simulink model "sampleModel1976_1_sub_sub"  (R2023a)
settings: Solver=VariableStepAuto  StartTime=0.0  StopTime=10.0  RelTol=1e-3
libraries: hdlsllib x5, simulink x1
settings Model: Creator=user1  LastModifiedBy=user1
settings OptimizationCC: BlockReduction=off  ConditionallyExecuteInputs=off

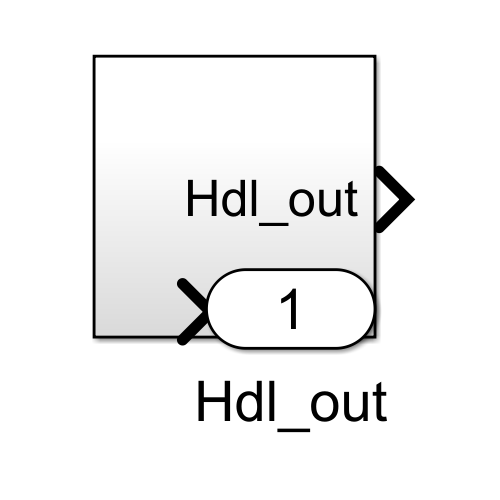
[thumbnail: Simulink's stored preview of the top-level diagram]
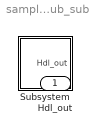
== system sampleModel1976_1_sub_sub ==
  Subsystem : Subsystem
  Hdl_out : Outport  OutDataTypeStr=uint8

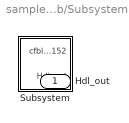
== system sampleModel1976_1_sub_sub/Subsystem ==
  Subsystem : Subsystem
  Hdl_out : Outport  OutDataTypeStr=uint8

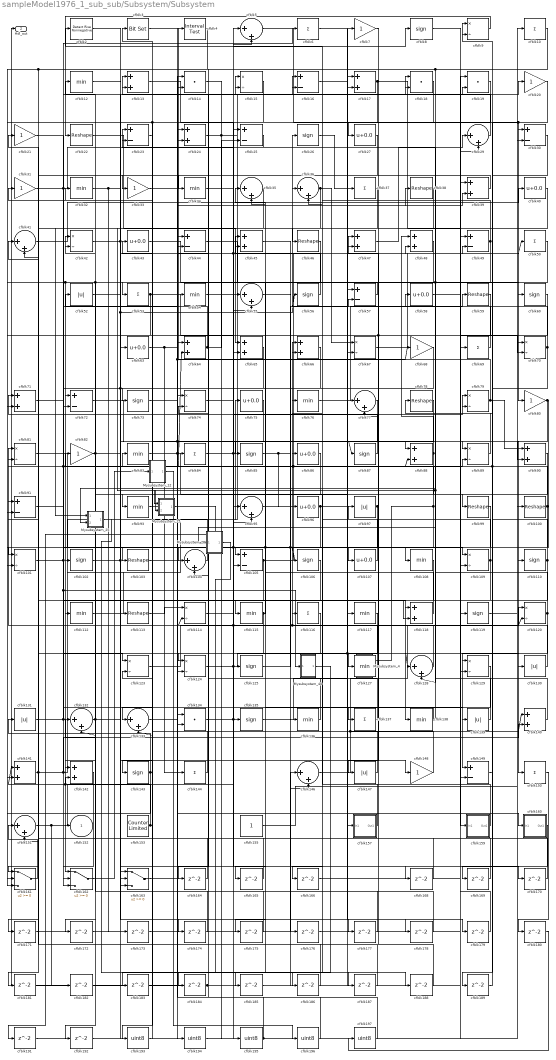
== system sampleModel1976_1_sub_sub/Subsystem/Subsystem ==
  Mysubsystem_12 : Subsystem  TreatAsAtomicUnit=on  RTWFcnName=Mysubsystem_12
      settings: RTWFcnNameOpts=User specified  RTWFileNameOpts=Use function name
  Mysubsystem_15 : Subsystem  TreatAsAtomicUnit=on  RTWFcnName=Mysubsystem_15
      settings: RTWFcnNameOpts=User specified  RTWFileNameOpts=Use function name
  Mysubsystem_25 : Subsystem  TreatAsAtomicUnit=on  RTWFcnName=Mysubsystem_25
      settings: RTWFcnNameOpts=User specified  RTWFileNameOpts=Use function name
  Mysubsystem_28 : Subsystem  TreatAsAtomicUnit=on  RTWFcnName=Mysubsystem_28
      settings: RTWFcnNameOpts=User specified  RTWFileNameOpts=Use function name
  Mysubsystem_4 : Subsystem  TreatAsAtomicUnit=on  RTWFcnName=Mysubsystem_4
      settings: RTWFcnNameOpts=User specified  RTWFileNameOpts=Use function name
  Mysubsystem_40 : Subsystem  TreatAsAtomicUnit=on  RTWFcnName=Mysubsystem_40
      settings: RTWFcnNameOpts=User specified  RTWFileNameOpts=Use function name
  cfblk{6,10,37,50,53,69,84,116,137,144,150} (11 alike) : Sum  Inputs=+  OutDataTypeStr=uint8
  cfblk{22,38,46,59,78,99..100,103,113} (9 alike) : Reshape
  cfblk{9,15,42,67,70,74,79,81,89,101,109,114,120,123..124,129} (16 alike) : Product  Inputs=*/  OutDataTypeStr=uint8  RndMeth=Zero  SaturateOnIntegerOverflow=on
  cfblk{8,26,56,60,73,85,87,102,106,110,119,125,135,143} (14 alike) : Signum
  cfblk{5,29,35..36,41,55,77,95,104,128,132..133,146,151} (14 alike) : Sum  Inputs=|++  OutDataTypeStr=uint8
  cfblk{16,23,25,30,44,49,57,72,91,105,149} (11 alike) : Sum  Inputs=+-  OutDataTypeStr=uint8
  cfblk{27,40,43,58,63,75,86,96,107} (9 alike) : Bias  Bias=0.0  SaturateOnIntegerOverflow=off
  cfblk{12,32,34,54,76,83,93,108,112,115,117,127,136,138} (14 alike) : MinMax  OutDataTypeStr=uint8
  cfblk{13,17,24,39,45,47..48,64..66,71,88,90,118,140..142} (17 alike) : Sum  OutDataTypeStr=uint8
  cfblk{52,97,130..131,139,147} (6 alike) : Abs  OutDataTypeStr=uint8  SaturateOnIntegerOverflow=off
  cfblk{14,18..19,134} (4 alike) : DotProduct  OutDataTypeStr=uint8
  cfblk{7,20..21,31,33,68,80,82,148} (9 alike) : Gain  OutDataTypeStr=uint8
  cfblk153 : hdlsllib/Sources/Counter Limited  uplimit=7  tsamp=-1
  cfblk155 : Constant  OutDataTypeStr=uint8  SampleTime=-1
  cfblk157 : Subsystem
      settings: LibrarySourceBlock=|
      | hdlsllib/Ports &
      | Subsystems/Subsystem
  cfblk159 : Subsystem
      settings: LibrarySourceBlock=|
      | hdlsllib/Ports &
      | Subsystems/Subsystem
  cfblk160 : Subsystem
      settings: LibrarySourceBlock=|
      | hdlsllib/Ports &
      | Subsystems/Subsystem
  cfblk161 : Switch  OutDataTypeStr=uint8  SaturateOnIntegerOverflow=off  InputSameDT=off
  cfblk162 : Switch  OutDataTypeStr=uint8  SaturateOnIntegerOverflow=off  InputSameDT=off
  cfblk163 : Switch  OutDataTypeStr=uint8  SaturateOnIntegerOverflow=off  InputSameDT=off
  cfblk{164..166,168..189,191..192} (27 alike) : Delay  SampleTime=1
  cfblk{193..197} (5 alike) : DataTypeConversion  OutDataTypeStr=uint8  SaturateOnIntegerOverflow=off  RndMeth=Floor
  cfblk2 : hdlsllib/Logic and Bit Operations/Detect Rise Nonnegative  vinit=0  OutDataTypeStr=uint8
  cfblk3 : simulink/Logic and Bit Operations/Bit Set  iBit=0
      settings: LibrarySourceBlock=|
      | hdlsllib/Logic and Bit
      | Operations/Bit Set
  cfblk4 : hdlsllib/Logic and Bit Operations/Interval Test  IntervalClosedRight=on  uplimit=0.5  IntervalClosedLeft=on  lowlimit=-0.5  OutDataTypeStr=uint8
  cfblk152 : Outport  OutDataTypeStr=uint8  VectorParamsAs1DForOutWhenUnconnected=off
  Hdl_out : Outport  Port=2  OutDataTypeStr=uint8
  wires:
  Mysubsystem_40/1(Out1) -> cfblk183/1
  Mysubsystem_28/1(Out1) -> cfblk188/1
  Mysubsystem_25/1(Out1) -> cfblk184/1
  Mysubsystem_15/1(Out1) -> cfblk191/1
  cfblk38/1 -> Mysubsystem_15/1(In1)
  Mysubsystem_12/1(Out1) -> cfblk196/1
  cfblk162/1 -> Mysubsystem_12/1(In1)
  Mysubsystem_4/1(Out1) -> cfblk21/1, cfblk143/1
  cfblk197/1 -> cfblk14/2
  cfblk180/1 -> cfblk197/1
  cfblk196/1 -> cfblk14/1
  cfblk195/1 -> cfblk104/2, cfblk100/1
  cfblk194/1 -> cfblk119/1
  cfblk3/1 -> cfblk194/1
  cfblk193/1 -> cfblk3/1
  cfblk77/1 -> cfblk193/1
  cfblk192/1 -> cfblk63/1
  cfblk191/1 -> cfblk95/2
  cfblk189/1 -> cfblk9/2
  cfblk188/1 -> cfblk47/2
  cfblk187/1 -> cfblk163/1
  cfblk186/1 -> cfblk81/2
  cfblk185/1 -> cfblk57/1
  cfblk184/1 -> cfblk65/2, Hdl_out/1
  cfblk183/1 -> cfblk146/1
  cfblk182/1 -> cfblk55/1
  cfblk181/1 -> cfblk19/1
  cfblk116/1 -> cfblk181/1
  cfblk150/1 -> cfblk180/1
  cfblk179/1 -> cfblk49/1
  cfblk178/1 -> cfblk134/1
  cfblk177/1 -> cfblk132/1
  cfblk176/1 -> cfblk77/1
  cfblk45/1 -> cfblk176/1
  cfblk175/1 -> cfblk163/2
  cfblk129/1 -> cfblk175/1
  cfblk174/1 -> cfblk42/2
  cfblk173/1 -> cfblk5/2
  cfblk172/1 -> cfblk149/2
  cfblk171/1 -> cfblk74/1
  cfblk170/1 -> cfblk44/1
  cfblk169/1 -> cfblk17/1
  cfblk160/1(Out1) -> cfblk169/1
  cfblk168/1 -> cfblk13/2
  cfblk166/1 -> cfblk29/2
  cfblk165/1 -> cfblk64/1
  cfblk164/1 -> cfblk41/1
  cfblk75/1 -> cfblk164/1
  cfblk2/1 -> cfblk88/1
  cfblk157/1(Out1) -> cfblk2/1
  cfblk12/1 -> cfblk113/1
  cfblk70/1 -> cfblk36/2, cfblk189/1
  cfblk136/1 -> cfblk44/2
  cfblk153/1 -> cfblk142/2, cfblk141/1, cfblk123/2
  cfblk59/1 -> cfblk147/1, cfblk172/1
  cfblk73/1 -> cfblk109/1
  cfblk133/1 -> cfblk49/2, cfblk68/1
  cfblk19/1 -> cfblk34/1
  cfblk58/1 -> cfblk70/2
  cfblk37/1 -> cfblk101/1
  cfblk161/1 -> cfblk151/1
  cfblk52/1 -> cfblk148/1
  cfblk43/1 -> cfblk60/1
  cfblk107/1 -> cfblk97/1
  cfblk138/1 -> Mysubsystem_28/1(In1), cfblk137/1
  cfblk66/1 -> cfblk105/1
  cfblk97/1 -> cfblk77/2, cfblk166/1
  cfblk125/1 -> cfblk57/2
  cfblk114/1 -> cfblk118/1
  cfblk32/1 -> cfblk173/1, cfblk174/1
  cfblk123/1 -> cfblk25/1, cfblk120/2
  cfblk57/1 -> cfblk53/1
  cfblk148/1 -> cfblk31/1
  cfblk124/1 -> cfblk130/1, cfblk89/2
  cfblk115/1 -> cfblk35/2, cfblk124/2
  cfblk40/1 -> cfblk46/1
  cfblk144/1 -> cfblk82/1
  cfblk103/1 -> cfblk160/1(In1)
  cfblk110/1 -> cfblk9/1, cfblk161/1
  cfblk102/1 -> cfblk56/1, cfblk19/2, cfblk177/1
  cfblk44/1 -> cfblk146/2
  cfblk67/1 -> cfblk30/2
  cfblk41/1 -> cfblk40/1
  cfblk49/1 -> cfblk85/1, cfblk16/2
  cfblk6/1 -> cfblk30/1
  cfblk21/1 -> cfblk123/1
  cfblk91/1 -> cfblk139/1
  cfblk23/1 -> cfblk73/1
  cfblk109/1 -> cfblk76/1, cfblk129/2
  cfblk80/1 -> cfblk110/1, cfblk90/2
  cfblk134/1 -> cfblk79/1, cfblk170/1
  cfblk68/1 -> cfblk72/2
  cfblk155/1 -> cfblk70/1
  cfblk53/1 -> cfblk71/2, cfblk95/1
  cfblk65/1 -> cfblk112/1, cfblk163/3
  cfblk139/1 -> cfblk23/1
  cfblk35/1 -> cfblk104/1
  cfblk13/1 -> cfblk55/2
  cfblk33/1 -> cfblk87/1, cfblk187/1
  cfblk93/1 -> cfblk48/2
  cfblk146/1 -> cfblk120/1, cfblk140/1
  cfblk141/1 -> cfblk86/1, cfblk140/2, cfblk91/1
  cfblk27/1 -> cfblk41/2
  cfblk25/1 -> cfblk24/2
  cfblk34/1 -> cfblk89/1
  cfblk56/1 -> cfblk45/1
  cfblk130/1 -> cfblk12/1
  cfblk137/1 -> cfblk74/2
  cfblk24/1 -> cfblk18/1, cfblk125/1
  cfblk127/1 -> cfblk66/2
  cfblk71/1 -> cfblk6/1
  cfblk4/1 -> cfblk91/2, cfblk171/1
  cfblk63/1 -> cfblk15/2, cfblk144/1
  cfblk106/1 -> cfblk115/1
  cfblk55/1 -> cfblk136/1
  cfblk30/1 -> cfblk99/1
  cfblk74/1 -> cfblk135/1
  cfblk142/1 -> cfblk162/3
  cfblk85/1 -> cfblk109/2, cfblk178/1, cfblk96/1
  cfblk18/1 -> cfblk67/2
  cfblk10/1 -> cfblk108/1, cfblk124/1
  cfblk90/1 -> cfblk102/1
  cfblk8/1 -> cfblk69/1
  cfblk46/1 -> cfblk84/1
  cfblk5/1 -> cfblk27/1
  cfblk132/1 -> cfblk42/1, cfblk168/1
  cfblk140/1 -> Mysubsystem_25/2(In2), Mysubsystem_15/2(In2)
  cfblk128/1 -> cfblk114/2, cfblk116/1
  cfblk7/1 -> cfblk127/1
  cfblk83/1 -> cfblk157/1(In1), cfblk39/2
  cfblk14/1 -> cfblk195/1
  cfblk87/1 -> cfblk71/1
  cfblk112/1 -> cfblk75/1
  cfblk95/1 -> cfblk7/1
  cfblk131/1 -> cfblk88/2, cfblk16/1, cfblk66/1
  cfblk147/1 -> cfblk32/1
  cfblk39/1 -> cfblk33/1
  cfblk105/1 -> cfblk47/1, cfblk39/1, cfblk151/2
  cfblk78/1 -> cfblk133/1
  cfblk17/1 -> cfblk133/2, cfblk101/2, cfblk159/1(In1)
  cfblk31/1 -> cfblk105/2, cfblk106/1, cfblk5/1, cfblk18/2
  cfblk108/1 -> cfblk138/1
  cfblk163/1 -> cfblk24/1
  cfblk117/1 -> cfblk162/2
  cfblk29/1 -> cfblk13/1
  cfblk119/1 -> cfblk10/1
  cfblk60/1 -> cfblk72/1
  cfblk100/1 -> cfblk64/2, cfblk79/2, cfblk141/2
  cfblk9/1 -> cfblk22/1
  cfblk54/1 -> cfblk36/1
  cfblk151/1 -> cfblk8/1, cfblk50/1, cfblk182/1
  cfblk120/1 -> cfblk149/1, cfblk58/1
  cfblk42/1 -> cfblk15/1, cfblk134/2
  cfblk118/1 -> cfblk35/1
  cfblk69/1 -> cfblk26/1
  cfblk64/1 -> cfblk52/1, cfblk25/2
  cfblk48/1 -> cfblk162/1, cfblk161/3, cfblk132/2
  cfblk149/1 -> cfblk81/1
  cfblk99/1 -> cfblk152/1, cfblk165/1
  cfblk15/1 -> cfblk103/1
  cfblk113/1 -> cfblk114/1
  cfblk16/1 -> cfblk117/1
  cfblk50/1 -> cfblk128/2, cfblk185/1
  cfblk20/1 -> cfblk80/1, cfblk129/1
  cfblk47/1 -> cfblk29/1
  cfblk135/1 -> cfblk17/2
  cfblk22/1 -> cfblk65/1
  cfblk36/1 -> Mysubsystem_25/1(In1), cfblk67/1
  cfblk104/1 -> cfblk43/1
  cfblk79/1 -> cfblk4/1, cfblk90/1
  cfblk96/1 -> cfblk128/1, cfblk179/1, cfblk142/1
  cfblk76/1 -> cfblk59/1
  cfblk86/1 -> cfblk93/1
  cfblk72/1 -> cfblk150/1
  cfblk81/1 -> cfblk107/1
  cfblk88/1 -> cfblk48/1, cfblk186/1
  cfblk89/1 -> cfblk78/1
  cfblk26/1 -> cfblk37/1
  cfblk143/1 -> cfblk131/1, cfblk23/2, cfblk161/2
  cfblk82/1 -> cfblk45/2, cfblk192/1
  cfblk84/1 -> cfblk20/1, cfblk38/1
  cfblk101/1 -> Mysubsystem_40/1(In1), cfblk118/2, cfblk54/1
  cfblk159/1(Out1) -> cfblk83/1

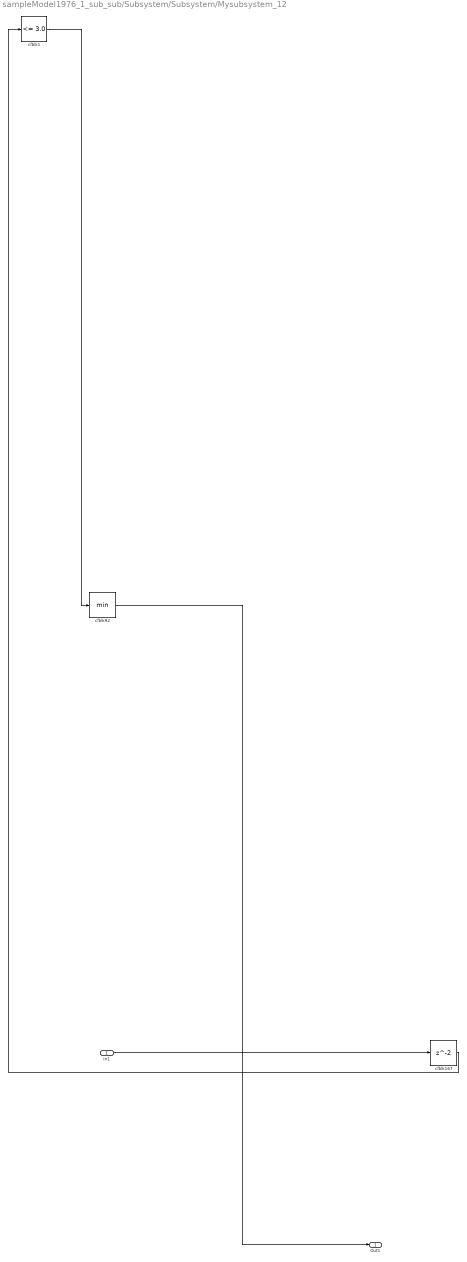
== system sampleModel1976_1_sub_sub/Subsystem/Subsystem/Mysubsystem_12 ==
  In1 : Inport
  cfblk1 : hdlsllib/Logic and Bit Operations/Compare To Constant  relop=<=  const=3.0  OutDataTypeStr=boolean
  cfblk167 : Delay  SampleTime=1
  cfblk92 : MinMax
  Out1 : Outport
  wires:
  cfblk1/1 -> cfblk92/1
  In1/1 -> cfblk167/1
  cfblk167/1 -> cfblk1/1
  cfblk92/1 -> Out1/1

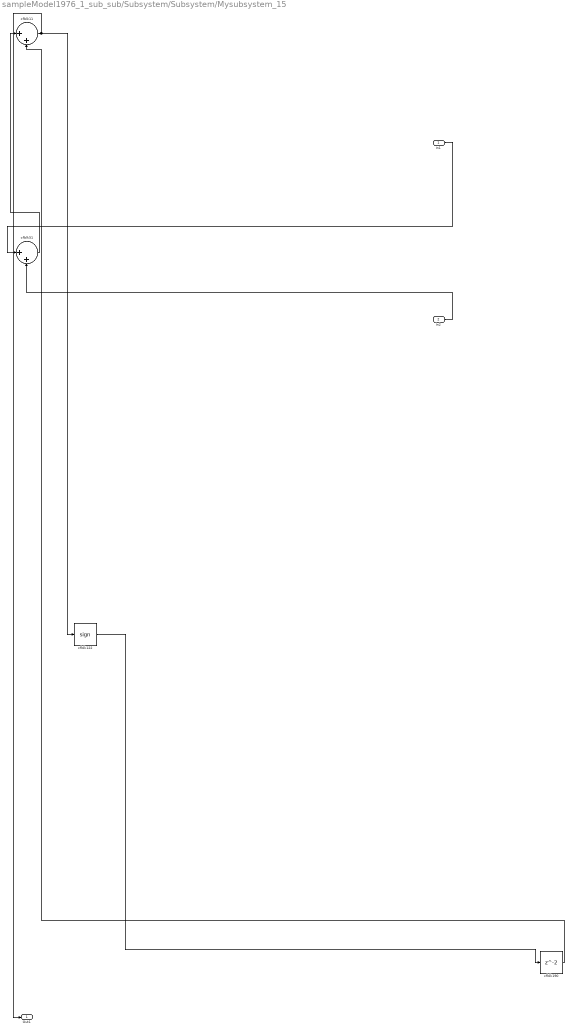
== system sampleModel1976_1_sub_sub/Subsystem/Subsystem/Mysubsystem_15 ==
  In1 : Inport
  In2 : Inport  Port=2
  cfblk11 : Sum  Inputs=|++
  cfblk122 : Signum
  cfblk190 : Delay  SampleTime=1
  cfblk51 : Sum  Inputs=|++
  Out1 : Outport
  wires:
  cfblk122/1 -> cfblk190/1
  cfblk51/1 -> cfblk11/1
  cfblk11/1 -> Out1/1, cfblk122/1
  In2/1 -> cfblk51/2
  cfblk190/1 -> cfblk11/2
  In1/1 -> cfblk51/1

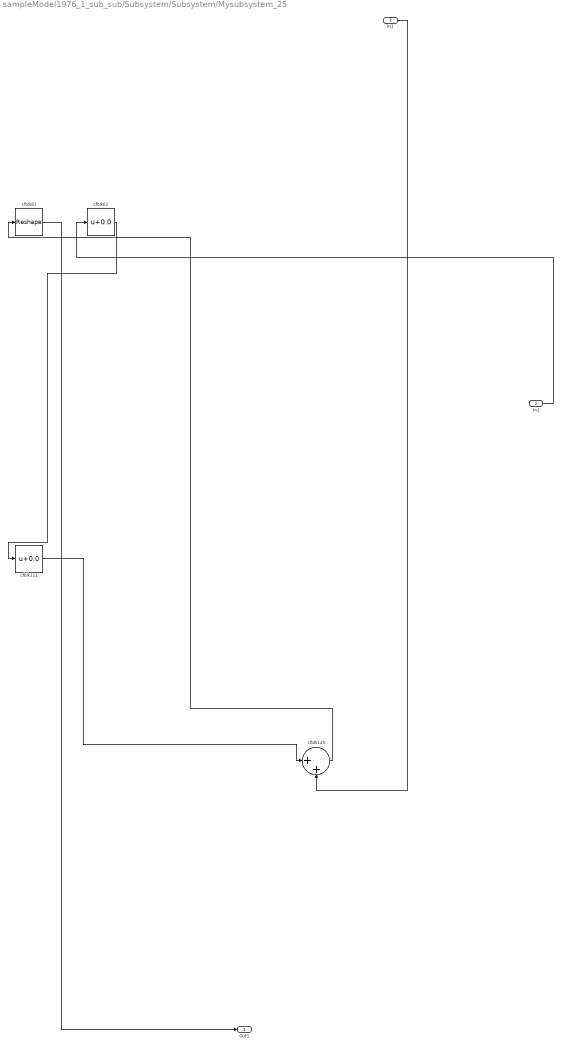
== system sampleModel1976_1_sub_sub/Subsystem/Subsystem/Mysubsystem_25 ==
  In1 : Inport
  In2 : Inport  Port=2
  cfblk111 : Bias  Bias=0.0  SaturateOnIntegerOverflow=off
  cfblk145 : Sum  Inputs=|++
  cfblk61 : Reshape
  cfblk62 : Bias  Bias=0.0  SaturateOnIntegerOverflow=off
  Out1 : Outport
  wires:
  cfblk145/1 -> cfblk61/1
  cfblk62/1 -> cfblk111/1
  In2/1 -> cfblk62/1
  cfblk111/1 -> cfblk145/1
  In1/1 -> cfblk145/2
  cfblk61/1 -> Out1/1

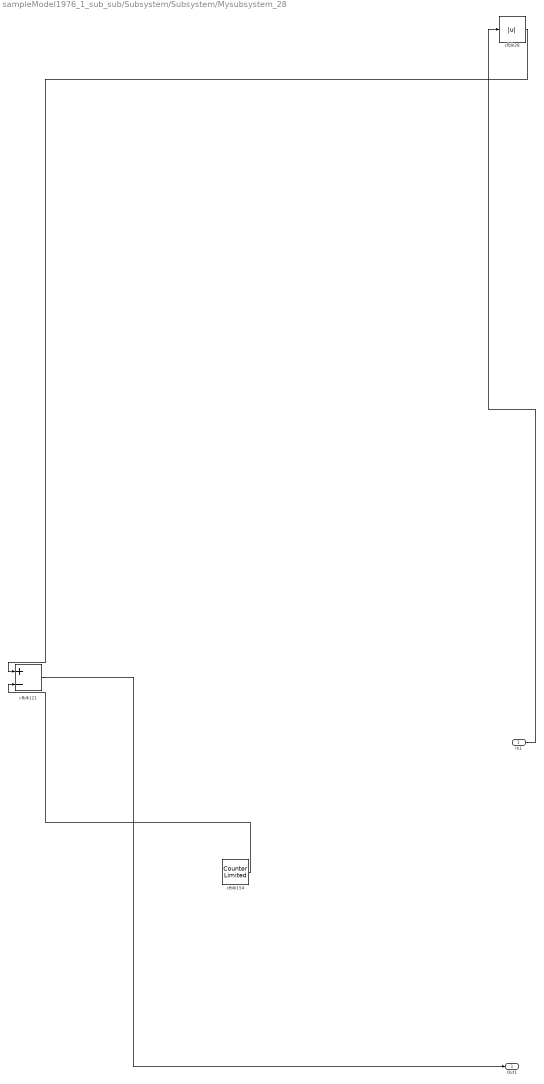
== system sampleModel1976_1_sub_sub/Subsystem/Subsystem/Mysubsystem_28 ==
  In1 : Inport
  cfblk121 : Sum  Inputs=+-
  cfblk154 : hdlsllib/Sources/Counter Limited  uplimit=7  tsamp=-1
  cfblk28 : Abs  SaturateOnIntegerOverflow=off
  Out1 : Outport
  wires:
  cfblk154/1 -> cfblk121/2
  cfblk28/1 -> cfblk121/1
  cfblk121/1 -> Out1/1
  In1/1 -> cfblk28/1

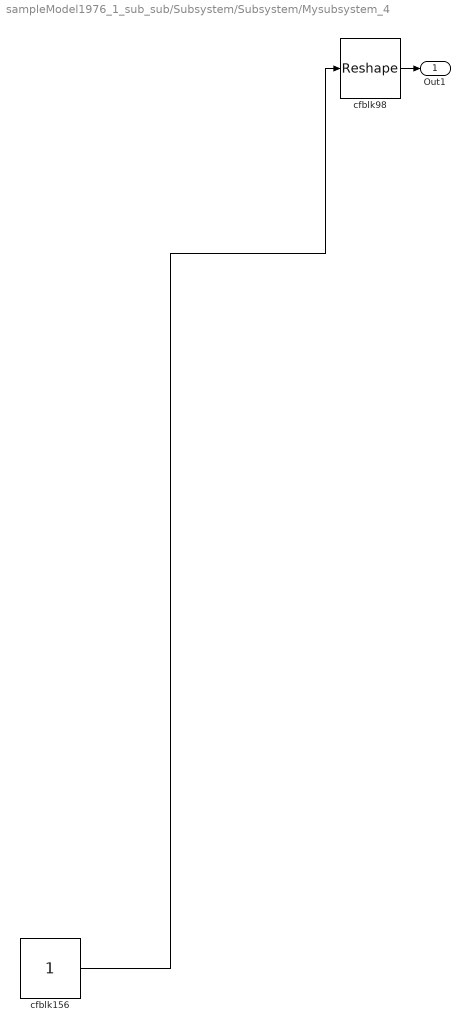
== system sampleModel1976_1_sub_sub/Subsystem/Subsystem/Mysubsystem_4 ==
  cfblk156 : Constant  SampleTime=-1
  cfblk98 : Reshape
  Out1 : Outport
  wires:
  cfblk156/1 -> cfblk98/1
  cfblk98/1 -> Out1/1

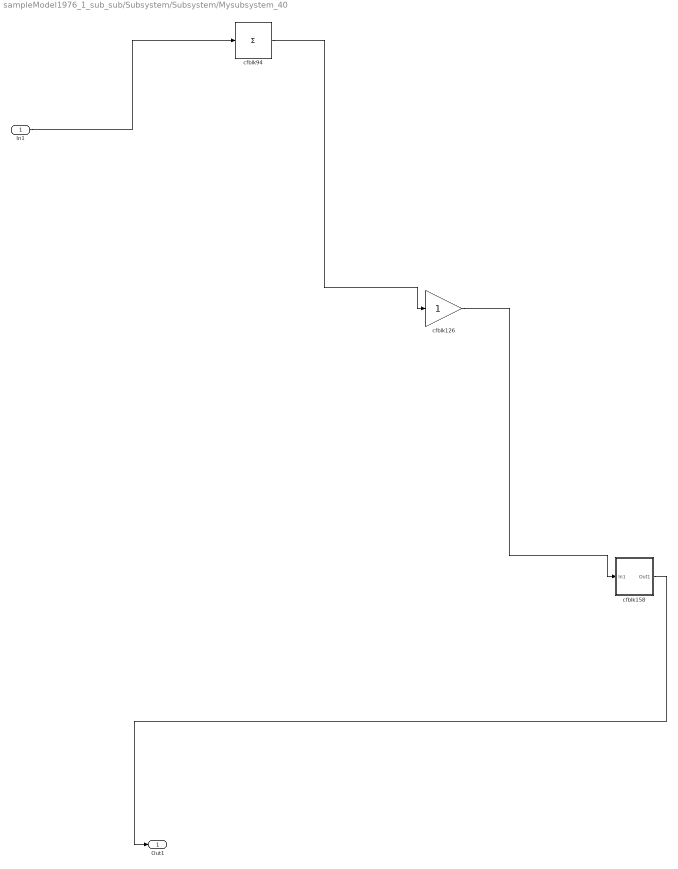
== system sampleModel1976_1_sub_sub/Subsystem/Subsystem/Mysubsystem_40 ==
  In1 : Inport
  cfblk126 : Gain
  cfblk158 : Subsystem
      settings: LibrarySourceBlock=|
      | hdlsllib/Ports &
      | Subsystems/Subsystem
  cfblk94 : Sum  Inputs=+
  Out1 : Outport
  wires:
  cfblk158/1(Out1) -> Out1/1
  cfblk94/1 -> cfblk126/1
  In1/1 -> cfblk94/1
  cfblk126/1 -> cfblk158/1(In1)

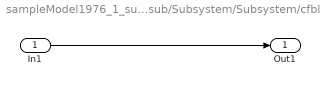
== system sampleModel1976_1_sub_sub/Subsystem/Subsystem/cfblk157 ==
  In1 : Inport
  Out1 : Outport
  wires:
  In1/1 -> Out1/1

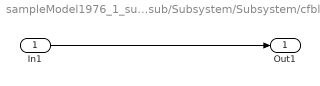
== system sampleModel1976_1_sub_sub/Subsystem/Subsystem/cfblk159 ==
  In1 : Inport
  Out1 : Outport
  wires:
  In1/1 -> Out1/1

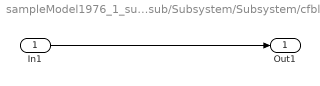
== system sampleModel1976_1_sub_sub/Subsystem/Subsystem/cfblk160 ==
  In1 : Inport
  Out1 : Outport
  wires:
  In1/1 -> Out1/1

== system sampleModel1976_1_sub_sub/Subsystem/Subsystem/Mysubsystem_40/cfblk158 ==
  In1 : Inport
  Out1 : Outport
  wires:
  In1/1 -> Out1/1
